simulink model "Write_LEDs"  (R2017a)
settings: Solver=ode2  StartTime=0.0  StopTime=inf  FixedStep=0.001  RelTol=1e-3  EnableMultiTasking=on
InitFcn:
  | set_param(gcs, 'ZoomFactor','FitSystem')
model workspace (MAT data in the model file):
  target_system = 1
undefined symbols (not defined in the file): HIL
libraries: quarc_library x3
settings Model: SimulationMode=external  ExtModeTrigDuration=10000  Creator=dmadill  LastModifiedBy=mbohra
settings SolverCC: PositivePriorityOrder=on
settings DataIOCC: LimitDataPoints=on  SaveFormat=Array
settings DebuggingCC: SolverPrmCheckMsg=warning  SFUnexpectedBacktrackingDiag=warning  SFNoUnconditionalDefaultTransitionDiag=warning  SFExecutionAtInitializationDiag=none
settings HardwareCC: ProdBitPerLong=64  ProdLargestAtomicFloat=None  ProdHWDeviceType=Intel->x86-64
settings ModelReferenceCC: PropagateSignalLabelsOutOfModel=off
settings RTWCC: SystemTargetFile=quarc_linux_duovero_2016.tlc  TemplateMakefile=quarc_linux_duovero_2016_tmf  Description=QUARC Linux DuoVero 2016 Target (QBall 2, QBot 2)
settings STFCustomTargetCC: TargetLibSuffix=.a  TargetPreCompLibLocation=C:\PROGRA~3\QUARC\lib\2017a\LI8355~1\release  ConcurrentExecutionCompliant=on  SystemTargetFile=quarc_linux_duovero_2016.tlc
settings GRTTargetCC: TargetLibSuffix=.a  TargetPreCompLibLocation=C:\PROGRA~3\QUARC\lib\2017a\LI8355~1\release  TargetLangStandard=C89/C90 (ANSI)  ParMdlRefBuildCompliant=off  CompOptLevelCompliant=off  CombineOutputUpdateFcns=off  MatFileLogging=off  CPPClassGenCompliant=off  GRTInterface=on  UseToolchainInfoCompliant=off  ExtMode=on  ExtModeMexFile=quarc_comm  ExtModeMexArgs='-w -d /tmp -uri %u','tcpip://192.168.2.x:17001'
settings ConfigComp: CovMetricSettings=dw  CovHtmlReporting=on  CovSaveCumulativeToWorkspaceVar=on  CovSaveSingleToWorkspaceVar=on  CovExternalEMLEnable=off  CovSFcnEnable=off

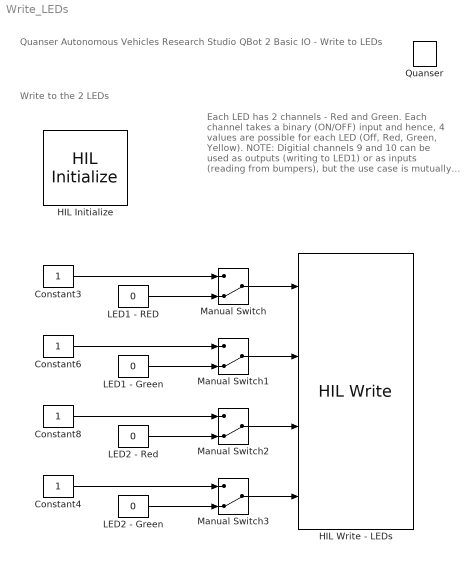
== system Write_LEDs ==
  note: Write to the 2 LEDs
  note: Quanser Autonomous Vehicles Research Studio
      | QBot 2 Basic IO - Write to LEDs
  note: Each LED has 2 channels - Red and Green. Each channel takes a binary (ON/OFF) input and hence, 4 values are possible for each LED (Off, Red, Green, Yellow).
      |
      | NOTE: Digitial channels 9 and 10 can be used as outputs (writing to LED1) or as inputs (reading from bumpers), but the use case is mutually exclusive. Thus, it is not possible to both write to LED1 and read from the bumpers simultaneously. Configure these channels to only do one of the 2 things. You can write to LED2 without restrictions via digital channels 11 and 12.
  Constant{3..4,6,8} (4 alike) : Constant
  HIL Initialize : quarc_library/Data Acquisition/Generic/Configuration/HIL Initialize  Priority=-99  object_name=HIL-1  board_type=qbot2  board_number=0  board_options=enc0_dir=0;enc0_filter=1;enc0_a=0;enc0_b=0;enc0_z=1;enc0_reload=0;enc1_dir=0;enc1_filter=1;enc1_a=0;enc1_b=0;enc1_z=1;enc1_reload=0;pwm0_immediate=0;pwm1_immediate=0;pwm2_immediate=0;pwm3_immediate=0;  exclusive=off  active=off  hardware_clocks=[]  clock_modes=[]  initial_clock_frequencies=[]  set_clock_params_at_start=off  set_clock_params_at_switch_in=off  set_clock_frequencies_at_start=off  set_clock_frequencies_at_switch_in=off  analog_input_channels=[0:9]  analog_input_configurations=[]  analog_input_maximums=[5 5 5 5 16.5 3.3 3.3 3.3 3.3]  analog_input_minimums=[0 0 0 0 0 0 0 0 0]  set_analog_input_params_at_start=off  set_analog_input_params_at_switch_in=off  analog_output_channels=[]  analog_output_maximums=[]  analog_output_minimums=[]  initial_analog_outputs=[]  final_analog_outputs=[]  watchdog_analog_outputs=[]  set_analog_output_params_at_start=off  set_analog_output_params_at_switch_in=off  set_analog_outputs_at_start=off  set_analog_outputs_at_switch_in=off  set_analog_outputs_at_terminate=off  set_analog_outputs_at_switch_out=off  set_analog_outputs_on_watchdog=off  digital_input_channels=[]  digital_output_channels=[9:12]  digital_output_configuration=[]  initial_digital_outputs=[0]  final_digital_outputs=[0]  watchdog_digital_outputs=[0]  set_digital_output_params_at_start=off  set_digital_output_params_at_switch_in=off  set_digital_outputs_at_start=on  set_digital_outputs_at_switch_in=off  set_digital_outputs_at_terminate=on  set_digital_outputs_at_switch_out=off  set_digital_outputs_on_watchdog=on  encoder_channels=[0:3]  quadrature=[4]  encoder_filter_frequency=[]  initial_encoder_counts=[0]  set_encoder_params_at_start=on  set_encoder_params_at_switch_in=off  set_encoder_counts_at_start=on  set_encoder_counts_at_switch_in=off  pwm_channels=[0:3]  pwm_modes=[0]  pwm_frequency=[20e6/1024]  pwm_configuration=[0]  pwm_alignment=[0]  pwm_polarity=[1]  pwm_leading_deadband=[0]  pwm_trailing_deadband=[0]  initial_pwm_outputs=[0]  final_pwm_outputs=[0]  watchdog_pwm_outputs=[0]  set_pwm_params_at_start=on  set_pwm_params_at_switch_in=off  set_pwm_outputs_at_start=on  set_pwm_outputs_at_switch_in=off  set_pwm_outputs_at_terminate=on  set_pwm_outputs_at_switch_out=off  set_pwm_outputs_on_watchdog=on  other_output_channels=[2000:2001 14000 16000]  initial_other_outputs=[0 0 0 7]  final_other_outputs=[0 0 0 7]  watchdog_other_outputs=[]  set_other_outputs_at_start=on  set_other_outputs_at_switch_in=off  set_other_outputs_at_terminate=on  set_other_outputs_at_switch_out=off  set_other_outputs_on_watchdog=off
  HIL Write - LEDs : quarc_library/Data Acquisition/Generic/Immediate I//O/HIL Write  object_name=HIL-1  analog_channels=[]  pwm_channels=[]  digital_channels=[9 10 11 12]  other_channels=[]  sample_time=-1  active=off  vector_input=off
  LED1 - Green : Constant  Value=0
  LED1 - RED : Constant  Value=0
  LED2 - Green : Constant  Value=0
  LED2 - Red : Constant  Value=0
  Manual Switch{,1..3} (4 alike) : ManualSwitch  CurrentSetting=0
  Quanser : quarc_library/Logos/Quanser
  wires:
  Constant6/1 -> Manual Switch1/1
  Manual Switch1/1 -> HIL Write - LEDs/2
  Constant8/1 -> Manual Switch2/1
  Manual Switch2/1 -> HIL Write - LEDs/3
  LED1 - Green/1 -> Manual Switch1/2
  Manual Switch/1 -> HIL Write - LEDs/1
  LED2 - Green/1 -> Manual Switch3/2
  Constant4/1 -> Manual Switch3/1
  LED1 - RED/1 -> Manual Switch/2
  Constant3/1 -> Manual Switch/1
  Manual Switch3/1 -> HIL Write - LEDs/4
  LED2 - Red/1 -> Manual Switch2/2
